simulink subsystem "NoSuspensionRear"  (R2025a)
settings: Solver=VariableStepAuto  StartTime=0.0  StopTime=10.0  RelTol=1e-3
undefined symbols (not defined in the file): PlntWhlNumFrnt
settings Model: ModifiedByFormat=The MathWorks, Inc.  Creator=The MathWorks, Inc.  LastModifiedBy=The MathWorks, Inc.
settings DebuggingCC: SubsystemReferenceDiagnosticForUnitTest=warning
settings RTWCC: GPUComputeCapability=3.5

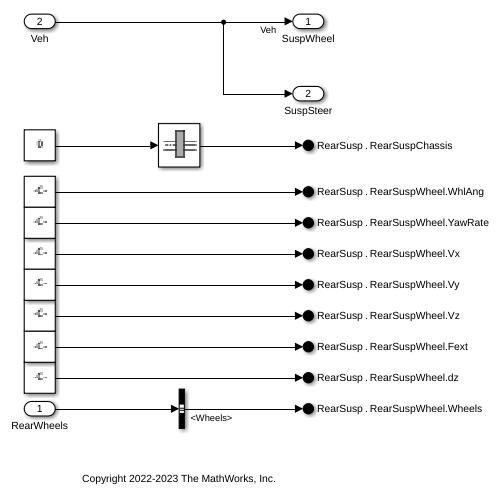
[thumbnail: Simulink's stored preview of the top-level diagram]
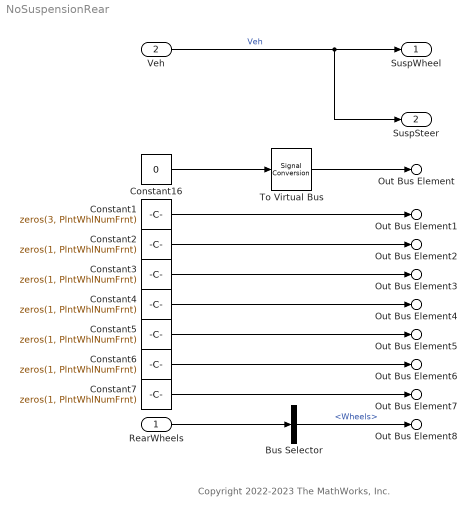
== system NoSuspensionRear ==
  note: Copyright 2022-2023 The MathWorks, Inc.
  RearWheels : Inport
  Veh : Inport  Port=2
  Bus Selector : BusSelector  OutputSignals=Wheels
  Constant1 : Constant  Value=zeros(3, PlntWhlNumFrnt)  SampleTime=Inf
  Constant16 : Constant  Value=0  OutDataTypeStr=Bus: RearSuspChassisBUS  SampleTime=Inf
  Constant{2..7} (6 alike) : Constant  Value=zeros(1, PlntWhlNumFrnt)  SampleTime=Inf
  To Virtual Bus : SignalConversion  ConversionOutput=Virtual bus  OverrideOpt=off
  SuspWheel : Outport
  SuspSteer : Outport  Port=2
  Out Bus Element : Outport  Port=3  PortName=RearSusp  Element=RearSuspChassis
  Out Bus Element1 : Outport  Port=3  PortName=RearSusp  Element=RearSuspWheel.WhlAng
  Out Bus Element2 : Outport  Port=3  PortName=RearSusp  Element=RearSuspWheel.YawRate
  Out Bus Element3 : Outport  Port=3  PortName=RearSusp  Element=RearSuspWheel.Vx
  Out Bus Element4 : Outport  Port=3  PortName=RearSusp  Element=RearSuspWheel.Vy
  Out Bus Element5 : Outport  Port=3  PortName=RearSusp  Element=RearSuspWheel.Vz
  Out Bus Element6 : Outport  Port=3  PortName=RearSusp  Element=RearSuspWheel.Fext
  Out Bus Element7 : Outport  Port=3  PortName=RearSusp  Element=RearSuspWheel.dz
  Out Bus Element8 : Outport  Port=3  PortName=RearSusp  Element=RearSuspWheel.Wheels
  wires:
  Constant5/1 -> Out Bus Element5/1
  Constant4/1 -> Out Bus Element4/1
  Constant1/1 -> Out Bus Element1/1
  Constant3/1 -> Out Bus Element3/1
  Constant7/1 -> Out Bus Element7/1
  Constant6/1 -> Out Bus Element6/1
  Constant2/1 -> Out Bus Element2/1
  Bus Selector/1 -> Out Bus Element8/1  "<Wheels>"
  RearWheels/1 -> Bus Selector/1
  To Virtual Bus/1 -> Out Bus Element/1
  Constant16/1 -> To Virtual Bus/1
  Veh/1 -> SuspWheel/1, SuspSteer/1  "Veh"
